simulink model "ACTLAB2SIMULINK_B220061"  (R2021b)
settings: Solver=VariableStepAuto  StartTime=0.0  StopTime=10.0  RelTol=1e-3
settings Model: Creator=mluser  LastModifiedBy=yash7

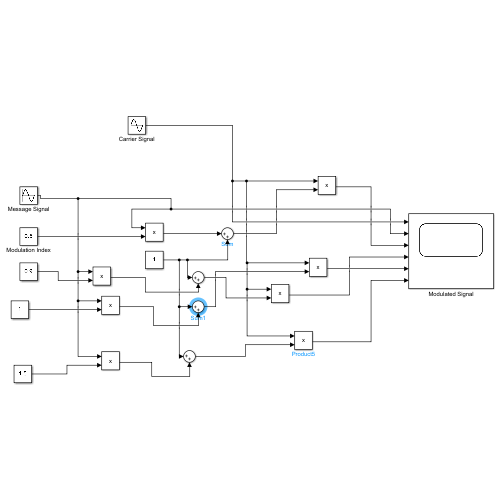
[thumbnail: Simulink's stored preview of the top-level diagram]
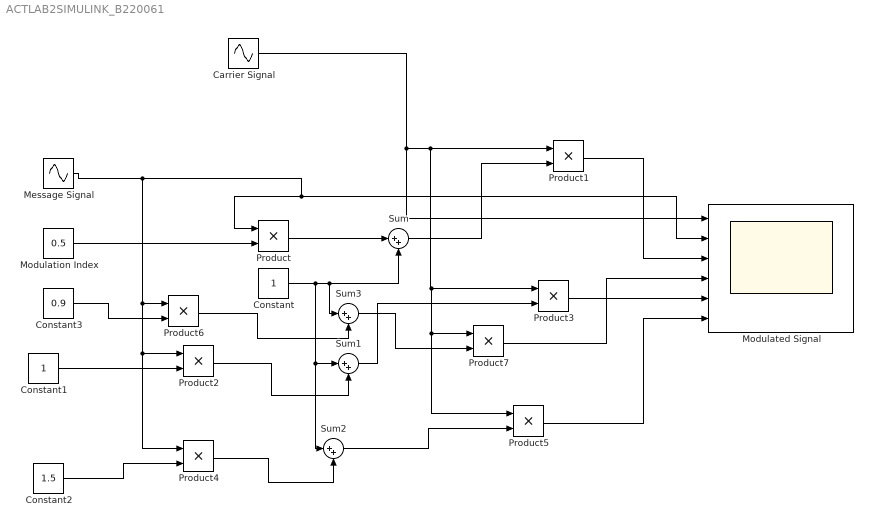
== system ACTLAB2SIMULINK_B220061 ==
  Carrier Signal : Sin  Frequency=50  SampleTime=0
  Constant : Constant
  Constant1 : Constant
  Constant2 : Constant  Value=1.5
  Constant3 : Constant  Value=0.9
  Message Signal : Sin  Frequency=2  SampleTime=0
  Modulated Signal : Scope  NumInputPorts=6
  Modulation Index : Constant  Value=0.5
  Product{,1..7} (8 alike) : Product
  Sum{,1..3} (4 alike) : Sum  Inputs=|++
  wires:
  Carrier Signal/1 -> Modulated Signal/1, Product7/1, Product5/1, Product3/1, Product1/1
  Message Signal/1 -> Product6/1, Product4/1, Product2/1, Product/1, Modulated Signal/2
  Modulation Index/1 -> Product/2
  Product/1 -> Sum/1
  Sum/1 -> Product1/2
  Constant/1 -> Sum2/1, Sum1/1, Sum3/1, Sum/2
  Product1/1 -> Modulated Signal/3
  Constant1/1 -> Product2/2
  Product2/1 -> Sum1/2
  Sum1/1 -> Product3/2
  Constant2/1 -> Product4/2
  Product4/1 -> Sum2/2
  Sum2/1 -> Product5/2
  Product5/1 -> Modulated Signal/6
  Product3/1 -> Modulated Signal/5
  Constant3/1 -> Product6/2
  Product6/1 -> Sum3/2
  Sum3/1 -> Product7/2
  Product7/1 -> Modulated Signal/4
